simulink model "SF011A_EotLrng"  (R2013b)
settings: Solver=FixedStepDiscrete  SolverMode=SingleTasking  StartTime=0.0  StopTime=1  FixedStep=0.002  RelTol=1e-3
values from neighbouring files (symbols this model uses):
  ARCHGLBPRM_FLOATZEROTHD_ULS_F32 = DataDict.Constant    [SF011A_EotLrng_DataDict.m]
  CNVTOMILLISEC_MILLISECPERCNT_F32 = DataDict.Constant    [SF011A_EotLrng_DataDict.m]
  CORRLNFLT_CNT_U08 = DataDict.Constant    [SF011A_EotLrng_DataDict.m]
  DEBSTEP_CNT_U16 = DataDict.Constant    [SF011A_EotLrng_DataDict.m]
  EOTLIMDETD_CNT_LOGL = DataDict.Constant    [SF011A_EotLrng_DataDict.m]
  EOTLIMNOTDETD_CNT_LOGL = DataDict.Constant    [SF011A_EotLrng_DataDict.m]
  EotLrngAuthyStrtLrn = DataDict.Calibration    [SF011A_EotLrng_DataDict.m]
  EotLrngEotLrnTmr = DataDict.Calibration    [SF011A_EotLrng_DataDict.m]
  EotLrngHwAgOverTrvlCnt = DataDict.Calibration    [SF011A_EotLrng_DataDict.m]
  EotLrngHwAgOverTrvlEntr = DataDict.Calibration    [SF011A_EotLrng_DataDict.m]
  EotLrngHwAgOverTrvlExit = DataDict.Calibration    [SF011A_EotLrng_DataDict.m]
  EotLrngHwTqEotLrn = DataDict.Calibration    [SF011A_EotLrng_DataDict.m]
  EotLrngMotVelEotLrn = DataDict.Calibration    [SF011A_EotLrng_DataDict.m]
  EotLrngRackTrvlMax = DataDict.Calibration    [SF011A_EotLrng_DataDict.m]
  EotLrngRackTrvlMin = DataDict.Calibration    [SF011A_EotLrng_DataDict.m]
  EotLrngRstAuthyMin = DataDict.Calibration    [SF011A_EotLrng_DataDict.m]
  EotProtnRackTrvlLimrEna = DataDict.ImprtdCal    [SF011A_EotLrng_DataDict.m]
  HwAgOverTrvl = DataDict.NTC    [SF011A_EotLrng_DataDict.m]
  HWAGOVERTRVLMAXCNT_CNT_U08 = DataDict.Constant    [SF011A_EotLrng_DataDict.m]
  NODEBSTEP_CNT_U16 = DataDict.Constant    [SF011A_EotLrng_DataDict.m]
  OUTOFRNGFLT_CNT_U08 = DataDict.Constant    [SF011A_EotLrng_DataDict.m]
  RackEotStorgFlt = DataDict.NTC    [SF011A_EotLrng_DataDict.m]
  SIGAVLFLT_CNT_U08 = DataDict.Constant    [SF011A_EotLrng_DataDict.m]
undefined symbols (not defined in the file or in its folder): NtcSts1, NvmGetErrSts1, SigQlfr1
libraries: simulink x19, NxtrNvM x12, NxtrAbslt x5, NxtrLim x4, NxtrMax x3, NxtrMin x3
(part 3 of 7)

== system SF011A_EotLrng/EotLrng/EotLrngInit1/NvmNotVal ==
  Action Port : ActionPort  ActionType=then
  Cal1 : Constant  RequirementInfo="{'linktype_rmi_doors' '0000ba59 (/E-STEER Core/SubSystem Specifications/Application Functions/SF011A Learned EOT Limits)' '#SF011A_124' 'true' 'REQ:  SF011A_124' '' } %GIDa_035de4f9_96cc_4fa1_acd4_8bfcce4812e0"  Value=EotLrngRackTrvlMin
  Cal2 : Constant  RequirementInfo="{'linktype_rmi_doors' '0000ba59 (/E-STEER Core/SubSystem Specifications/Application Functions/SF011A Learned EOT Limits)' '#SF011A_124' 'true' 'REQ:  SF011A_124' '' } %GIDa_01b27a86_f72b_45a9_877f_2950e2d94a2a"  Value=EotLrngRackTrvlMin
  Constant1 : Constant  RequirementInfo="{'linktype_rmi_doors' '0000ba59 (/E-STEER Core/SubSystem Specifications/Application Functions/SF011A Learned EOT Limits)' '#SF011A_124' 'true' 'REQ:  SF011A_124' '' } %GIDa_1ebed793_de7b_4df7_85c2_e94d2e34449d"  Value=EOTLIMNOTDETD_CNT_LOGL
  Constant2 : Constant  RequirementInfo="{'linktype_rmi_doors' '0000ba59 (/E-STEER Core/SubSystem Specifications/Application Functions/SF011A Learned EOT Limits)' '#SF011A_124' 'true' 'REQ:  SF011A_124' '' } %GIDa_066674ad_e74a_483b_a55d_646f85c07109"  Value=EOTLIMNOTDETD_CNT_LOGL
  CopyRight2 : Subsystem  Description=|  mask(Copyright Information){none=on}
      | Copyright info block.                                               
      |                                                                     
      | Place copyright information at the top of every subsystem in design.
      mask prompts: none "No parameters"
      mask help: Place copyright information at the top of every subsystem in design.
      mask Display:
      | NxtrConf = 'Nexteer Confidential';
      | 
      | sys = bdroot; %handle for the current model ("system")
      | first = get_param(sys,'Created');
      | if(isempty(first))
      |     first = datestr(now,'yyyy');
      | else
      |     first = first(end-3:end);  %year is last four digits
      | end
      | 
      | last = get_param(sys,'LastModifiedDate');
      | if isempty(last)
      |     last = datestr(now,'yyyy');
      | else
      |     last = last(end-3:end);
      | end
      | 
      | if strcmp(first,last)
      |     fprintf('%s -- Copyright %s Nexteer',NxtrConf,first)
      | else
      |     fprintf('%s -- %s%s- %s Nexteer',NxtrConf,char(169),first,last)
      | end
  EotNotDetd : DataStoreWrite  RequirementInfo="{'linktype_rmi_doors' '0000ba59 (/E-STEER Core/SubSystem Specifications/Application Functions/SF011A Learned EOT Limits)' '#SF011A_124' 'true' 'REQ:  SF011A_124' '' } %GIDa_67ea3644_1ed5_47b1_a1b5_07943d39ffbc"  DataStoreName=EotNvmData  DataStoreElements=EotNvmData.CwEot#EotNvmData.CcwEot#EotNvmData.CwEotDetd#EotNvmData.CcwEotDetd
  Set Ram Block Status : NxtrNvM/Set Ram Block Status  RequirementInfo="{'linktype_rmi_doors' '0000ba59 (/E-STEER Core/SubSystem Specifications/Application Functions/SF011A Learned EOT Limits)' '#SF011A_124' 'true' 'REQ:  SF011A_124' '' } %GIDa_cd84de67_5aef_4c01_bda0_51f502c42aea"  FuncName=Set Ram Block Status  NvMBlockName=EotNvmData  VoidFuncRtn=on  BlockChanged_DSN=NvMSRBS_BlockChanged1  Return_DSN=NvMSRBS_Return1
      settings: AttributesFormatString=%<FuncName>
  Unary Minus : UnaryMinus  RequirementInfo="{'linktype_rmi_doors' '0000ba59 (/E-STEER Core/SubSystem Specifications/Application Functions/SF011A Learned EOT Limits)' '#SF011A_124' 'true' 'REQ:  SF011A_124' '' } %GIDa_d2217dbc_c775_4562_a13a_db7a1fc359c1"
  WriteFlag : Constant  RequirementInfo="{'linktype_rmi_doors' '0000ba59 (/E-STEER Core/SubSystem Specifications/Application Functions/SF011A Learned EOT Limits)' '#SF011A_124' 'true' 'REQ:  SF011A_124' '' } %GIDa_0fcbdb88_2c6a_4773_b445_1f58a3cfa24b"  OutDataTypeStr=boolean
      settings: AttributesFormatString=%<OutDataTypeStr>
  wires:
  Cal1/1 -> EotNotDetd/1
  Constant2/1 -> EotNotDetd/3
  Constant1/1 -> EotNotDetd/4
  Cal2/1 -> Unary Minus/1
  Unary Minus/1 -> EotNotDetd/2
  WriteFlag/1 -> Set Ram Block Status/1

== system SF011A_EotLrng/EotLrng/EotLrngInit1/RstEot ==
  note: 'ResetLimitRequest' is applicable only when SRL Enable is FALSE.
      | So 'IF' block is executed only when 'EotProtnRackTrvlLimrEna' is FALSE.
  Action Port : ActionPort  ActionType=then
  Cal1 : Constant  RequirementInfo="{'linktype_rmi_doors' '0000ba59 (/E-STEER Core/SubSystem Specifications/Application Functions/SF011A Learned EOT Limits)' '#SF011A_65' 'true' 'REQ:  SF011A_65' '' } %GIDa_8a14116a_f5ff_4f97_ae11_7182dd2cd95a"  Value=EotLrngRackTrvlMin
  Cal2 : Constant  RequirementInfo="{'linktype_rmi_doors' '0000ba59 (/E-STEER Core/SubSystem Specifications/Application Functions/SF011A Learned EOT Limits)' '#SF011A_66' 'true' 'REQ:  SF011A_66' '' } %GIDa_f5c0a088_5e82_430d_9c85_3e33e4dedd97"  Value=EotLrngRackTrvlMin
  Calibration4 : Constant  Value=EotProtnRackTrvlLimrEna
  ChkRstLimReq : Subsystem  RequirementInfo="{'linktype_rmi_doors' '0000ba59 (/E-STEER Core/SubSystem Specifications/Application Functions/SF011A Learned EOT Limits)' '#SF011A_120' 'true' 'REQ:  SF011A_120' '' } %GIDa_b83ed28f_298f_4fb9_b00a_69d67f564ffe"  TreatAsAtomicUnit=on
  Constant2 : Constant  RequirementInfo="{'linktype_rmi_doors' '0000ba59 (/E-STEER Core/SubSystem Specifications/Application Functions/SF011A Learned EOT Limits)' '#SF011A_67' 'true' 'REQ:  SF011A_67' '' } %GIDa_aa357eb7_da8e_4d45_9211_17e2d7de8510"  Value=EOTLIMNOTDETD_CNT_LOGL
  Constant3 : Constant  RequirementInfo="{'linktype_rmi_doors' '0000ba59 (/E-STEER Core/SubSystem Specifications/Application Functions/SF011A Learned EOT Limits)' '#SF011A_68' 'true' 'REQ:  SF011A_68' '' } %GIDa_8e713c15_fb38_440b_b663_257e60f908ef"  Value=EOTLIMNOTDETD_CNT_LOGL
  Copyright1 : Subsystem  Description=|  mask(Copyright Information){none=on}
      | Copyright info block.                                               
      |                                                                     
      | Place copyright information at the top of every subsystem in design.
      mask prompts: none "No parameters"
      mask help: Place copyright information at the top of every subsystem in design.
      mask Display:
      | NxtrConf = 'Nexteer Confidential';
      | 
      | sys = bdroot; %handle for the current model ("system")
      | first = get_param(sys,'Created');
      | if(isempty(first))
      |     first = datestr(now,'yyyy');
      | else
      |     first = first(end-3:end);  %year is last four digits
      | end
      | 
      | last = get_param(sys,'LastModifiedDate');
      | if isempty(last)
      |     last = datestr(now,'yyyy');
      | else
      |     last = last(end-3:end);
      | end
      | 
      | if strcmp(first,last)
      |     fprintf('%s\nCopyright  %s Nexteer',NxtrConf,first);
      | else
      |     fprintf('%s\n%s%s-%s Nexteer',NxtrConf,char(169),first,last);
      | end
  EotNotDetd : DataStoreWrite  RequirementInfo="{'linktype_rmi_doors' '0000ba59 (/E-STEER Core/SubSystem Specifications/Application Functions/SF011A Learned EOT Limits)' '#SF011A_65' 'true' 'REQ:  SF011A_65' '' ; 'linktype_rmi_doors' '0000ba59 (/E-STEER Core/SubSystem Specifications/Application Functions/SF011A Learned EOT Limits)' '#SF011A_66' 'true' 'REQ:  SF011A_66' '' ; 'linktype_rmi_doors' '0000ba59 (/E-STEER Core/SubSystem Specifications/Application Functions/SF011A Learned EOT Limits)' '#SF011A_67' 'true' 'REQ:  SF011A_67' '' ; 'linktype_rmi_doors' '0000ba59 (/E-STEER Core/SubSystem Specifications/Application Functions/SF011A Learned EOT Limits)' '#SF011A_68' 'true' 'REQ:  SF011A_68' '' } %GIDa_c154dafa_482c_4d0d_b49a_45c1c207fc69"  DataStoreName=EotNvmData  DataStoreElements=EotNvmData.CwEot#EotNvmData.CcwEot#EotNvmData.CwEotDetd#EotNvmData.CcwEotDetd
  If1 : If  IfExpression=~u1  ShowElse=off
  Unary Minus : UnaryMinus  RequirementInfo="{'linktype_rmi_doors' '0000ba59 (/E-STEER Core/SubSystem Specifications/Application Functions/SF011A Learned EOT Limits)' '#SF011A_66' 'true' 'REQ:  SF011A_66' '' } %GIDa_7d675248_4626_4542_a80b_dcf5738ed4de"
  wires:
  Cal1/1 -> EotNotDetd/1
  Constant2/1 -> EotNotDetd/3
  Constant3/1 -> EotNotDetd/4
  Cal2/1 -> Unary Minus/1
  Unary Minus/1 -> EotNotDetd/2
  Calibration4/1 -> If1/1
  If1/1 -> ChkRstLimReq/Action

== system SF011A_EotLrng/EotLrng/EotLrngInit1/SRLNotEna ==
  Action Port : ActionPort  ActionType=then
  CopyRight2 : Subsystem  Description=|  mask(Copyright Information){none=on}
      | Copyright info block.                                               
      |                                                                     
      | Place copyright information at the top of every subsystem in design.
      mask prompts: none "No parameters"
      mask help: Place copyright information at the top of every subsystem in design.
      mask Display:
      | NxtrConf = 'Nexteer Confidential';
      | 
      | sys = bdroot; %handle for the current model ("system")
      | first = get_param(sys,'Created');
      | if(isempty(first))
      |     first = datestr(now,'yyyy');
      | else
      |     first = first(end-3:end);  %year is last four digits
      | end
      | 
      | last = get_param(sys,'LastModifiedDate');
      | if isempty(last)
      |     last = datestr(now,'yyyy');
      | else
      |     last = last(end-3:end);
      | end
      | 
      | if strcmp(first,last)
      |     fprintf('%s -- Copyright %s Nexteer',NxtrConf,first)
      | else
      |     fprintf('%s -- %s%s- %s Nexteer',NxtrConf,char(169),first,last)
      | end
  Data Store Write1 : DataStoreWrite  RequirementInfo="{'linktype_rmi_doors' '0000ba59 (/E-STEER Core/SubSystem Specifications/Application Functions/SF011A Learned EOT Limits)' '#SF011A_125' 'true' 'REQ:  SF011A_125' '' } %GIDa_d378e069_f629_4d72_894b_869d827cea0f"  DataStoreName=CwEotRefTmr
  Data Store Write2 : DataStoreWrite  RequirementInfo="{'linktype_rmi_doors' '0000ba59 (/E-STEER Core/SubSystem Specifications/Application Functions/SF011A Learned EOT Limits)' '#SF011A_125' 'true' 'REQ:  SF011A_125' '' } %GIDa_c50f2ed6_18b8_4a79_9256_efd4e1cd0e04"  DataStoreName=CcwEotRefTmr
  GetRefTmr100MicroSec32bit : Subsystem  RequirementInfo="{'linktype_rmi_doors' '0000ba59 (/E-STEER Core/SubSystem Specifications/Application Functions/SF011A Learned EOT Limits)' '#SF011A_125' 'true' 'REQ:  SF011A_125' '' } %GIDa_8d57e8b2_6972_45c8_8aed_33e94bb589a0"
  Set Ram Block Status : NxtrNvM/Set Ram Block Status  RequirementInfo="{'linktype_rmi_doors' '0000ba59 (/E-STEER Core/SubSystem Specifications/Application Functions/SF011A Learned EOT Limits)' '#SF011A_71' 'true' 'REQ:  SF011A_71' '' } %GIDa_8d0a3400_ce1c_4c12_9bc7_eab84e420ace"  FuncName=Set Ram Block Status  NvMBlockName=EotNvmData  VoidFuncRtn=on  BlockChanged_DSN=NvMSRBS_BlockChanged2  Return_DSN=NvMSRBS_Return2
      settings: AttributesFormatString=%<FuncName>
  WriteFlag : Constant  RequirementInfo="{'linktype_rmi_doors' '0000ba59 (/E-STEER Core/SubSystem Specifications/Application Functions/SF011A Learned EOT Limits)' '#SF011A_71' 'true' 'REQ:  SF011A_71' '' } %GIDa_d9597664_5da8_4eef_8b58_6fe14386c65c"  OutDataTypeStr=boolean
      settings: AttributesFormatString=%<OutDataTypeStr>
  wires:
  GetRefTmr100MicroSec32bit/1(RefTmr) -> Data Store Write2/1, Data Store Write1/1
  WriteFlag/1 -> Set Ram Block Status/1

== system SF011A_EotLrng/EotLrng/EotLrngInit1/SetOverTrvlDiagcPass ==
  NtcNr : Inport
  NtcStInfo : Inport  Port=2
  NtcSts : Inport  Port=3
  DebStep : Inport  Port=4
  SetNtcSts : Subsystem  RequirementInfo={} %GIDa_9e323aaf_8c1e_43be_a15a_0107c73abfe9  TreatAsAtomicUnit=on
      settings: RTWSystemCode=Inline
  wires:
  NtcNr/1 -> SetNtcSts/1(NtcNr)  "NtcNr"
  NtcSts/1 -> SetNtcSts/3(NtcSts)
  DebStep/1 -> SetNtcSts/4(DebStep)
  NtcStInfo/1 -> SetNtcSts/2(NtcStInfo)

== system SF011A_EotLrng/EotLrng/EotLrngPer1/CopyRight2 ==

== system SF011A_EotLrng/EotLrng/EotLrngPer1/HwAgCwAndCcwMax ==
  HwAg : Inport  RequirementInfo={} %GIDa_58741c58_0ee8_47f7_8539_fc4bf25b9bfb
  HwAgAuthy : Inport  RequirementInfo="{'linktype_rmi_doors' '0000ba59 (/E-STEER Core/SubSystem Specifications/Application Functions/SF011A Learned EOT Limits)' '#SF011A_156' 'true' 'REQ:  SF011A_156' '' ; 'linktype_rmi_doors' '0000ba59 (/E-STEER Core/SubSystem Specifications/Application Functions/SF011A Learned EOT Limits)' '#SF011A_158' 'true' 'REQ:  SF011A_158' '' } %GIDa_fbd8c566_5363_4a96_8e79_d2f0f22f358c"  Port=2
  HwAgCwDetd : Inport  RequirementInfo={} %GIDa_42146e60_6491_4cfb_867f_f1091c71a37f  Port=3
  HwAgCcwDetd : Inport  RequirementInfo={} %GIDa_3f214823_f21d_45f8_844e_ba7a8ea07747  Port=4
  Conf : Sum  RequirementInfo="{'linktype_rmi_doors' '0000ba59 (/E-STEER Core/SubSystem Specifications/Application Functions/SF011A Learned EOT Limits)' '#SF011A_145' 'true' 'REQ:  SF011A_145' '' ; 'linktype_rmi_doors' '0000ba59 (/E-STEER Core/SubSystem Specifications/Application Functions/SF011A Learned EOT Limits)' '#SF011A_156' 'true' 'REQ:  SF011A_156' '' ; 'linktype_rmi_doors' '0000ba59 (/E-STEER Core/SubSystem Specifications/Application Functions/SF011A Learned EOT Limits)' '#SF011A_158' 'true' 'REQ:  SF011A_158' '' } %GIDa_bf8efe5e_d1fb_49c5_9ca8_3a5e9fe4b02d"  Inputs=+-
  Constant : Constant  RequirementInfo="{'linktype_rmi_doors' '0000ba59 (/E-STEER Core/SubSystem Specifications/Application Functions/SF011A Learned EOT Limits)' '#SF011A_156' 'true' 'REQ:  SF011A_156' '' ; 'linktype_rmi_doors' '0000ba59 (/E-STEER Core/SubSystem Specifications/Application Functions/SF011A Learned EOT Limits)' '#SF011A_158' 'true' 'REQ:  SF011A_158' '' } %GIDa_0eba6ba2_6b16_45eb_a7cf_ae1f1a9ed1c4"  OutDataTypeStr=single
      settings: AttributesFormatString=%<OutDataTypeStr>
  Constant4 : Constant  RequirementInfo="{'linktype_rmi_doors' '0000ba59 (/E-STEER Core/SubSystem Specifications/Application Functions/SF011A Learned EOT Limits)' '#SF011A_156' 'true' 'REQ:  SF011A_156' '' ; 'linktype_rmi_doors' '0000ba59 (/E-STEER Core/SubSystem Specifications/Application Functions/SF011A Learned EOT Limits)' '#SF011A_158' 'true' 'REQ:  SF011A_158' '' } %GIDa_d72fb292_81de_491b_ad99_a4a5661cf7d7"  Value=ARCHGLBPRM_FLOATZEROTHD_ULS_F32
  CopyRight2 : Subsystem  Description=|  mask(Copyright Information){none=on}
      | Copyright info block.                                               
      |                                                                     
      | Place copyright information at the top of every subsystem in design.
      mask prompts: none "No parameters"
      mask help: Place copyright information at the top of every subsystem in design.
      mask Display:
      | NxtrConf = 'Nexteer Confidential';
      | 
      | sys = bdroot; %handle for the current model ("system")
      | first = get_param(sys,'Created');
      | if(isempty(first))
      |     first = datestr(now,'yyyy');
      | else
      |     first = first(end-3:end);  %year is last four digits
      | end
      | 
      | last = get_param(sys,'LastModifiedDate');
      | if isempty(last)
      |     last = datestr(now,'yyyy');
      | else
      |     last = last(end-3:end);
      | end
      | 
      | if strcmp(first,last)
      |     fprintf('%s -- Copyright %s Nexteer',NxtrConf,first)
      | else
      |     fprintf('%s -- %s%s- %s Nexteer',NxtrConf,char(169),first,last)
      | end
  HwAgCwAndCcw : Subsystem  RequirementInfo="{'linktype_rmi_doors' '0000ba59 (/E-STEER Core/SubSystem Specifications/Application Functions/SF011A Learned EOT Limits)' '#SF011A_158' 'true' 'REQ:  SF011A_158' '' } %GIDa_77bc3317_1f5b_4708_9123_1bb25581bbdf"  TreatAsAtomicUnit=on
  If : If  RequirementInfo="{'linktype_rmi_doors' '0000ba59 (/E-STEER Core/SubSystem Specifications/Application Functions/SF011A Learned EOT Limits)' '#SF011A_156' 'true' 'REQ:  SF011A_156' '' ; 'linktype_rmi_doors' '0000ba59 (/E-STEER Core/SubSystem Specifications/Application Functions/SF011A Learned EOT Limits)' '#SF011A_158' 'true' 'REQ:  SF011A_158' '' } %GIDa_feff3a4a_5231_4460_af4d_ff321ace2938"  IfExpression=u1  ShowElse=off
  Relational Operator1 : RelationalOperator  RequirementInfo="{'linktype_rmi_doors' '0000ba59 (/E-STEER Core/SubSystem Specifications/Application Functions/SF011A Learned EOT Limits)' '#SF011A_156' 'true' 'REQ:  SF011A_156' '' ; 'linktype_rmi_doors' '0000ba59 (/E-STEER Core/SubSystem Specifications/Application Functions/SF011A Learned EOT Limits)' '#SF011A_158' 'true' 'REQ:  SF011A_158' '' } %GIDa_5f57789c_cdb5_4887_9bd9_e5225cc82d4e"  Operator=<  OutDataTypeStr=boolean
  wires:
  HwAg/1 -> HwAgCwAndCcw/1(HwAg)
  Conf/1 -> Relational Operator1/1
  Constant4/1 -> Relational Operator1/2
  Relational Operator1/1 -> If/1
  If/1 -> HwAgCwAndCcw/Action
  Constant/1 -> Conf/1
  HwAgAuthy/1 -> Conf/2
  HwAgCwDetd/1 -> HwAgCwAndCcw/2(HwAgCwDetd)
  HwAgCcwDetd/1 -> HwAgCwAndCcw/3(HwAgCcwDetd)

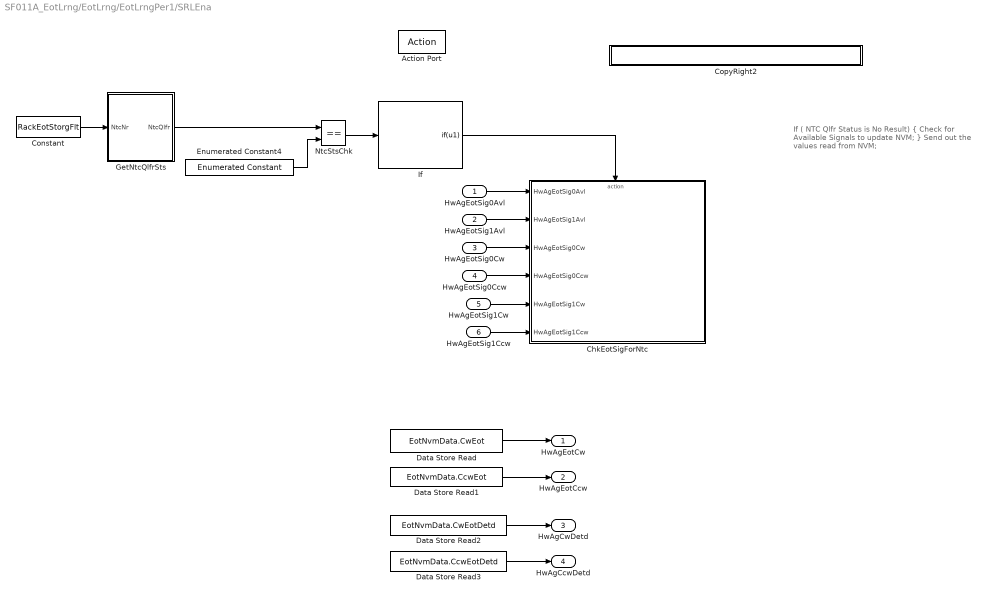
== system SF011A_EotLrng/EotLrng/EotLrngPer1/SRLEna ==
  note: If ( NTC Qlfr Status is No Result)
      | {
      | 	Check for Available Signals to update NVM;
      | }
      |
      | Send out the values read from NVM;
  HwAgEotSig0Avl : Inport
  HwAgEotSig1Avl : Inport  Port=2
  HwAgEotSig0Cw : Inport  Port=3
  HwAgEotSig0Ccw : Inport  Port=4
  HwAgEotSig1Cw : Inport  Port=5
  HwAgEotSig1Ccw : Inport  Port=6
  Action Port : ActionPort  ActionType=else
  ChkEotSigForNtc : Subsystem  Priority=2  TreatAsAtomicUnit=on
  Constant : Constant  Value=RackEotStorgFlt
  CopyRight2 : Subsystem  Description=|  mask(Copyright Information){none=on}
      | Copyright info block.                                               
      |                                                                     
      | Place copyright information at the top of every subsystem in design.
      mask prompts: none "No parameters"
      mask help: Place copyright information at the top of every subsystem in design.
      mask Display:
      | NxtrConf = 'Nexteer Confidential';
      | 
      | sys = bdroot; %handle for the current model ("system")
      | first = get_param(sys,'Created');
      | if(isempty(first))
      |     first = datestr(now,'yyyy');
      | else
      |     first = first(end-3:end);  %year is last four digits
      | end
      | 
      | last = get_param(sys,'LastModifiedDate');
      | if isempty(last)
      |     last = datestr(now,'yyyy');
      | else
      |     last = last(end-3:end);
      | end
      | 
      | if strcmp(first,last)
      |     fprintf('%s -- Copyright %s Nexteer',NxtrConf,first)
      | else
      |     fprintf('%s -- %s%s- %s Nexteer',NxtrConf,char(169),first,last)
      | end
  Data Store Read : DataStoreRead  RequirementInfo="{'linktype_rmi_doors' '0000ba59 (/E-STEER Core/SubSystem Specifications/Application Functions/SF011A Learned EOT Limits)' '#SF011A_151' 'true' 'REQ:  SF011A_151' '' } %GIDa_491bb231_a96c_471a_a0b1_cb46d3ab7fd8"  DataStoreName=EotNvmData  DataStoreElements=EotNvmData.CwEot
  Data Store Read1 : DataStoreRead  RequirementInfo="{'linktype_rmi_doors' '0000ba59 (/E-STEER Core/SubSystem Specifications/Application Functions/SF011A Learned EOT Limits)' '#SF011A_151' 'true' 'REQ:  SF011A_151' '' } %GIDa_e22716e1_ea90_4526_a8a2_524f602455ba"  DataStoreName=EotNvmData  DataStoreElements=EotNvmData.CcwEot
  Data Store Read2 : DataStoreRead  RequirementInfo="{'linktype_rmi_doors' '0000ba59 (/E-STEER Core/SubSystem Specifications/Application Functions/SF011A Learned EOT Limits)' '#SF011A_152' 'true' 'REQ:  SF011A_152' '' } %GIDa_803dbdde_f1bc_4dcd_811b_135296056d76"  DataStoreName=EotNvmData  DataStoreElements=EotNvmData.CwEotDetd
  Data Store Read3 : DataStoreRead  RequirementInfo="{'linktype_rmi_doors' '0000ba59 (/E-STEER Core/SubSystem Specifications/Application Functions/SF011A Learned EOT Limits)' '#SF011A_152' 'true' 'REQ:  SF011A_152' '' } %GIDa_81638686_3894_4a3b_89e5_bc8caeb35295"  DataStoreName=EotNvmData  DataStoreElements=EotNvmData.CcwEotDetd
  Enumerated Constant4 : simulink/Sources/Enumerated Constant  RequirementInfo="{'linktype_rmi_doors' '0000ba59 (/E-STEER Core/SubSystem Specifications/Application Functions/SF011A Learned EOT Limits)' '#SF011A_144' 'true' 'REQ:  SF011A_144' '' } %GIDa_d54fdf58_b16f_405c_be57_dbc33b57e03e"  OutDataTypeStr=Enum: SigQlfr1  Value=SigQlfr1.SIGQLFR_NORES  SampleTime=inf
  GetNtcQlfrSts : Subsystem  RequirementInfo="{'linktype_rmi_doors' '0000ba59 (/E-STEER Core/SubSystem Specifications/Application Functions/SF011A Learned EOT Limits)' '#SF011A_144' 'true' 'REQ:  SF011A_144' '' } %GIDa_4c60277e_e0ab_4449_8203_11119612fe69"  Priority=0  TreatAsAtomicUnit=on  mask(GetNTC){}
      mask help: GetNTC library block
      settings: RTWSystemCode=Inline
  If : If  RequirementInfo="{'linktype_rmi_doors' '0000ba59 (/E-STEER Core/SubSystem Specifications/Application Functions/SF011A Learned EOT Limits)' '#SF011A_144' 'true' 'REQ:  SF011A_144' '' } %GIDa_00dfac98_a167_441c_a0ad_0ab30e5da204"  Priority=1  IfExpression=u1  ShowElse=off
  NtcStsChk : RelationalOperator  RequirementInfo="{'linktype_rmi_doors' '0000ba59 (/E-STEER Core/SubSystem Specifications/Application Functions/SF011A Learned EOT Limits)' '#SF011A_144' 'true' 'REQ:  SF011A_144' '' } %GIDa_ddf88f27_8f18_4c5d_9adb_9f4c149e8d0b"  Operator===  OutDataTypeStr=boolean
  HwAgEotCw : Outport  RequirementInfo="{'linktype_rmi_doors' '0000ba59 (/E-STEER Core/SubSystem Specifications/Application Functions/SF011A Learned EOT Limits)' '#SF011A_151' 'true' 'REQ:  SF011A_151' '' } %GIDa_fda7daf0_aaae_4096_9ebe_71b9db7e29f8"
  HwAgEotCcw : Outport  RequirementInfo="{'linktype_rmi_doors' '0000ba59 (/E-STEER Core/SubSystem Specifications/Application Functions/SF011A Learned EOT Limits)' '#SF011A_151' 'true' 'REQ:  SF011A_151' '' } %GIDa_84ec16c1_5dae_46bb_8c56_2a910f1f9ddc"  Port=2
  HwAgCwDetd : Outport  RequirementInfo="{'linktype_rmi_doors' '0000ba59 (/E-STEER Core/SubSystem Specifications/Application Functions/SF011A Learned EOT Limits)' '#SF011A_152' 'true' 'REQ:  SF011A_152' '' } %GIDa_67f65cbe_992b_48c5_9d00_546aabda8cbc"  Port=3
  HwAgCcwDetd : Outport  RequirementInfo="{'linktype_rmi_doors' '0000ba59 (/E-STEER Core/SubSystem Specifications/Application Functions/SF011A Learned EOT Limits)' '#SF011A_152' 'true' 'REQ:  SF011A_152' '' } %GIDa_23fcd4ad_b638_4e85_88df_027c5135ac77"  Port=4
  wires:
  Constant/1 -> GetNtcQlfrSts/1(NtcNr)
  Enumerated Constant4/1 -> NtcStsChk/2
  NtcStsChk/1 -> If/1
  HwAgEotSig0Avl/1 -> ChkEotSigForNtc/1(HwAgEotSig0Avl)
  HwAgEotSig1Avl/1 -> ChkEotSigForNtc/2(HwAgEotSig1Avl)
  HwAgEotSig0Cw/1 -> ChkEotSigForNtc/3(HwAgEotSig0Cw)
  HwAgEotSig0Ccw/1 -> ChkEotSigForNtc/4(HwAgEotSig0Ccw)
  HwAgEotSig1Cw/1 -> ChkEotSigForNtc/5(HwAgEotSig1Cw)
  HwAgEotSig1Ccw/1 -> ChkEotSigForNtc/6(HwAgEotSig1Ccw)
  If/1 -> ChkEotSigForNtc/Action
  GetNtcQlfrSts/1(NtcQlfr) -> NtcStsChk/1
  Data Store Read2/1 -> HwAgCwDetd/1
  Data Store Read3/1 -> HwAgCcwDetd/1
  Data Store Read/1 -> HwAgEotCw/1
  Data Store Read1/1 -> HwAgEotCcw/1

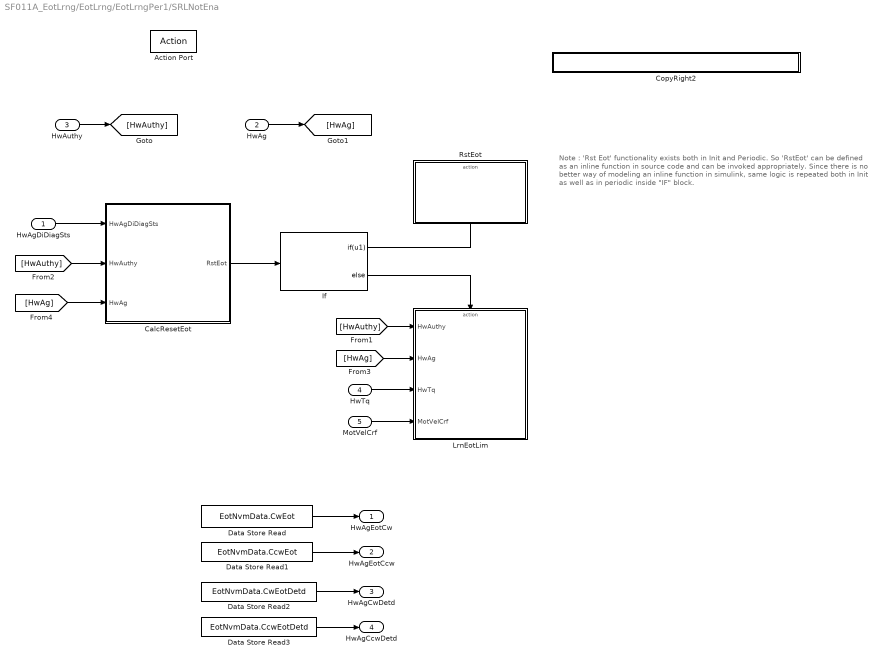
== system SF011A_EotLrng/EotLrng/EotLrngPer1/SRLNotEna ==
  note: Note : 'Rst Eot' functionality exists both in Init and Periodic.
      | So 'RstEot' can be defined as an inline function in source code and can be invoked
      | appropriately. Since there is no better way of modeling an inline function in simulink,
      | same logic is repeated both in Init as well as in periodic inside "IF" block.
  HwAgDiDiagSts : Inport
  HwAg : Inport  Port=2
  HwAuthy : Inport  Port=3
  HwTq : Inport  Port=4
  MotVelCrf : Inport  Port=5
  Action Port : ActionPort  ActionType=then
  CalcResetEot : Subsystem  Priority=0  TreatAsAtomicUnit=on
  CopyRight2 : Subsystem  Description=|  mask(Copyright Information){none=on}
      | Copyright info block.                                               
      |                                                                     
      | Place copyright information at the top of every subsystem in design.
      mask prompts: none "No parameters"
      mask help: Place copyright information at the top of every subsystem in design.
      mask Display:
      | NxtrConf = 'Nexteer Confidential';
      | 
      | sys = bdroot; %handle for the current model ("system")
      | first = get_param(sys,'Created');
      | if(isempty(first))
      |     first = datestr(now,'yyyy');
      | else
      |     first = first(end-3:end);  %year is last four digits
      | end
      | 
      | last = get_param(sys,'LastModifiedDate');
      | if isempty(last)
      |     last = datestr(now,'yyyy');
      | else
      |     last = last(end-3:end);
      | end
      | 
      | if strcmp(first,last)
      |     fprintf('%s -- Copyright %s Nexteer',NxtrConf,first)
      | else
      |     fprintf('%s -- %s%s- %s Nexteer',NxtrConf,char(169),first,last)
      | end
  Data Store Read : DataStoreRead  RequirementInfo="{'linktype_rmi_doors' '0000ba59 (/E-STEER Core/SubSystem Specifications/Application Functions/SF011A Learned EOT Limits)' '#SF011A_152' 'true' 'REQ:  SF011A_152' '' } %GIDa_e6e4a090_8f56_4550_9411_905043d89ec9"  DataStoreName=EotNvmData  DataStoreElements=EotNvmData.CwEot
  Data Store Read1 : DataStoreRead  RequirementInfo="{'linktype_rmi_doors' '0000ba59 (/E-STEER Core/SubSystem Specifications/Application Functions/SF011A Learned EOT Limits)' '#SF011A_152' 'true' 'REQ:  SF011A_152' '' } %GIDa_57f7b2c9_ce66_4e64_aa00_2e33be35bf96"  DataStoreName=EotNvmData  DataStoreElements=EotNvmData.CcwEot
  Data Store Read2 : DataStoreRead  RequirementInfo="{'linktype_rmi_doors' '0000ba59 (/E-STEER Core/SubSystem Specifications/Application Functions/SF011A Learned EOT Limits)' '#SF011A_152' 'true' 'REQ:  SF011A_152' '' } %GIDa_1c8ac1be_b2fe_42d3_9f1e_87bea7bc78f5"  DataStoreName=EotNvmData  DataStoreElements=EotNvmData.CwEotDetd
  Data Store Read3 : DataStoreRead  RequirementInfo="{'linktype_rmi_doors' '0000ba59 (/E-STEER Core/SubSystem Specifications/Application Functions/SF011A Learned EOT Limits)' '#SF011A_152' 'true' 'REQ:  SF011A_152' '' } %GIDa_fbf998d0_abbd_4e2e_9173_7ac660a7097a"  DataStoreName=EotNvmData  DataStoreElements=EotNvmData.CcwEotDetd
  If : If  RequirementInfo="{'linktype_rmi_doors' '0000ba59 (/E-STEER Core/SubSystem Specifications/Application Functions/SF011A Learned EOT Limits)' '#SF011A_77' 'true' 'REQ:  SF011A_77' '' } %GIDa_0aa79ea6_77ec_4eb1_817b_135a8ab293c6"  Priority=1  IfExpression=u1
  LrnEotLim : Subsystem  TreatAsAtomicUnit=on
  RstEot : Subsystem  RequirementInfo="{'linktype_rmi_doors' '0000ba59 (/E-STEER Core/SubSystem Specifications/Application Functions/SF011A Learned EOT Limits)' '#SF011A_64' 'true' 'REQ:  SF011A_64' '' ; 'linktype_rmi_doors' '0000ba59 (/E-STEER Core/SubSystem Specifications/Application Functions/SF011A Learned EOT Limits)' '#SF011A_77' 'true' 'REQ:  SF011A_77' '' } %GIDa_52c91bf7_5122_422c_9233_27632b93939a"  TreatAsAtomicUnit=on
  HwAgEotCw : Outport  RequirementInfo="{'linktype_rmi_doors' '0000ba59 (/E-STEER Core/SubSystem Specifications/Application Functions/SF011A Learned EOT Limits)' '#SF011A_152' 'true' 'REQ:  SF011A_152' '' } %GIDa_f2d57ba9_aa8d_479c_9cc8_16e180750fa0"
  HwAgEotCcw : Outport  RequirementInfo="{'linktype_rmi_doors' '0000ba59 (/E-STEER Core/SubSystem Specifications/Application Functions/SF011A Learned EOT Limits)' '#SF011A_152' 'true' 'REQ:  SF011A_152' '' } %GIDa_27db5f88_6347_4271_b0df_6a54758f3e06"  Port=2
  HwAgCwDetd : Outport  RequirementInfo="{'linktype_rmi_doors' '0000ba59 (/E-STEER Core/SubSystem Specifications/Application Functions/SF011A Learned EOT Limits)' '#SF011A_152' 'true' 'REQ:  SF011A_152' '' } %GIDa_b05d0ec9_37ec_4da9_bb3b_3c23aee6b93b"  Port=3
  HwAgCcwDetd : Outport  RequirementInfo="{'linktype_rmi_doors' '0000ba59 (/E-STEER Core/SubSystem Specifications/Application Functions/SF011A Learned EOT Limits)' '#SF011A_152' 'true' 'REQ:  SF011A_152' '' } %GIDa_425014ec_6d0c_4dba_84fc_301e2e49fc38"  Port=4
  wires:
  HwAuthy/1 -> [HwAuthy]
  If/1 -> RstEot/Action
  HwAgDiDiagSts/1 -> CalcResetEot/1(HwAgDiDiagSts)
  [HwAg] -> CalcResetEot/3(HwAg)
  CalcResetEot/1(RstEot) -> If/1
  [HwAuthy] -> CalcResetEot/2(HwAuthy)
  If/2 -> LrnEotLim/Action
  HwTq/1 -> LrnEotLim/3(HwTq)
  MotVelCrf/1 -> LrnEotLim/4(MotVelCrf)
  [HwAuthy] -> LrnEotLim/1(HwAuthy)
  HwAg/1 -> [HwAg]
  [HwAg] -> LrnEotLim/2(HwAg)
  Data Store Read2/1 -> HwAgCwDetd/1
  Data Store Read3/1 -> HwAgCcwDetd/1
  Data Store Read/1 -> HwAgEotCw/1
  Data Store Read1/1 -> HwAgEotCcw/1

== system SF011A_EotLrng/EotLrng/GetHwAgOverTrvlCnt/CopyRight2 ==

== system SF011A_EotLrng/EotLrng/RstHwAgOverTrvlCnt/CopyRight2 ==

== system SF011A_EotLrng/EotLrng/RstMaxHwAgCwAndCcw/CopyRight2 ==

== system SF011A_EotLrng/EotLrng/RtnMaxHwAgCwAndCcw/CopyRight2 ==

== system SF011A_EotLrng/EotLrng/SerlComRstEot/CopyRight2 ==

== system SF011A_EotLrng/EotLrng/SerlComRstEot/SetRstLimReq ==
  Action Port : ActionPort  ActionType=then
  Constant : Constant  RequirementInfo="{'linktype_rmi_doors' '0000ba59 (/E-STEER Core/SubSystem Specifications/Application Functions/SF011A Learned EOT Limits)' '#SF011A_123' 'true' 'REQ:  SF011A_123' '' } %GIDa_80072151_4aff_45b9_8875_461114410ad3"  Value=true  OutDataTypeStr=boolean
      settings: AttributesFormatString=%<OutDataTypeStr>
  CopyRight2 : Subsystem  Description=|  mask(Copyright Information){none=on}
      | Copyright info block.                                               
      |                                                                     
      | Place copyright information at the top of every subsystem in design.
      mask prompts: none "No parameters"
      mask help: Place copyright information at the top of every subsystem in design.
      mask Display:
      | NxtrConf = 'Nexteer Confidential';
      | 
      | sys = bdroot; %handle for the current model ("system")
      | first = get_param(sys,'Created');
      | if(isempty(first))
      |     first = datestr(now,'yyyy');
      | else
      |     first = first(end-3:end);  %year is last four digits
      | end
      | 
      | last = get_param(sys,'LastModifiedDate');
      | if isempty(last)
      |     last = datestr(now,'yyyy');
      | else
      |     last = last(end-3:end);
      | end
      | 
      | if strcmp(first,last)
      |     fprintf('%s -- Copyright %s Nexteer',NxtrConf,first)
      | else
      |     fprintf('%s -- %s%s- %s Nexteer',NxtrConf,char(169),first,last)
      | end
  Update PIM3 : DataStoreWrite  RequirementInfo="{'linktype_rmi_doors' '0000ba59 (/E-STEER Core/SubSystem Specifications/Application Functions/SF011A Learned EOT Limits)' '#SF011A_123' 'true' 'REQ:  SF011A_123' '' } %GIDa_a977ed3a_c109_468e_8bf0_813090a9fca0"  DataStoreName=RstLimReq
  wires:
  Constant/1 -> Update PIM3/1

== system SF011A_EotLrng/EotLrng/SetHwAgOverTrvlCnt/CopyRight2 ==

== system SF011A_EotLrng/EotLrng/EotLrngInit1/NvmNotOk/CopyRight2 ==

== system SF011A_EotLrng/EotLrng/EotLrngInit1/NvmNotVal/CopyRight2 ==

== system SF011A_EotLrng/EotLrng/EotLrngInit1/RstEot/ChkRstLimReq ==
  Action Port : ActionPort  ActionType=then
  CopyRight2 : Subsystem  Description=|  mask(Copyright Information){none=on}
      | Copyright info block.                                               
      |                                                                     
      | Place copyright information at the top of every subsystem in design.
      mask prompts: none "No parameters"
      mask help: Place copyright information at the top of every subsystem in design.
      mask Display:
      | NxtrConf = 'Nexteer Confidential';
      | 
      | sys = bdroot; %handle for the current model ("system")
      | first = get_param(sys,'Created');
      | if(isempty(first))
      |     first = datestr(now,'yyyy');
      | else
      |     first = first(end-3:end);  %year is last four digits
      | end
      | 
      | last = get_param(sys,'LastModifiedDate');
      | if isempty(last)
      |     last = datestr(now,'yyyy');
      | else
      |     last = last(end-3:end);
      | end
      | 
      | if strcmp(first,last)
      |     fprintf('%s -- Copyright %s Nexteer',NxtrConf,first)
      | else
      |     fprintf('%s -- %s%s- %s Nexteer',NxtrConf,char(169),first,last)
      | end
  Data Store Read4 : DataStoreRead  RequirementInfo="{'linktype_rmi_doors' '0000ba59 (/E-STEER Core/SubSystem Specifications/Application Functions/SF011A Learned EOT Limits)' '#SF011A_120' 'true' 'REQ:  SF011A_120' '' } %GIDa_bbdcaebb_aa54_4c32_aceb_dfb7e5459836"  DataStoreName=RstLimReq
  If : If  RequirementInfo="{'linktype_rmi_doors' '0000ba59 (/E-STEER Core/SubSystem Specifications/Application Functions/SF011A Learned EOT Limits)' '#SF011A_120' 'true' 'REQ:  SF011A_120' '' } %GIDa_0c4f3b6a_a79f_4beb_a24b_d33f2f2aabe0"  IfExpression=u1  ShowElse=off
  ResetLimReq : Subsystem  RequirementInfo="{'linktype_rmi_doors' '0000ba59 (/E-STEER Core/SubSystem Specifications/Application Functions/SF011A Learned EOT Limits)' '#SF011A_120' 'true' 'REQ:  SF011A_120' '' } %GIDa_2dbe23da_3ce9_4548_9ac3_4137e2e9edeb"  TreatAsAtomicUnit=on
  wires:
  Data Store Read4/1 -> If/1
  If/1 -> ResetLimReq/Action

== system SF011A_EotLrng/EotLrng/EotLrngInit1/RstEot/Copyright1 ==

== system SF011A_EotLrng/EotLrng/EotLrngInit1/SRLNotEna/CopyRight2 ==

== system SF011A_EotLrng/EotLrng/EotLrngInit1/SRLNotEna/GetRefTmr100MicroSec32bit ==
  note: 1 count = 100 uSec
  note: seconds
  note: microseconds
  note: counts
  note: Wrap-to-zero
  note: GetRefTmr100MicroSec32bit
  CopyRight2 : Subsystem  Description=|  mask(Copyright Information){none=on}
      | Copyright info block.                                               
      |                                                                     
      | Place copyright information at the top of every subsystem in design.
      mask prompts: none "No parameters"
      mask help: Place copyright information at the top of every subsystem in design.
      mask Display:
      | NxtrConf = 'Nexteer Confidential';
      | 
      | sys = bdroot; %handle for the current model ("system")
      | first = get_param(sys,'Created');
      | if(isempty(first))
      |     first = datestr(now,'yyyy');
      | else
      |     first = first(end-3:end);  %year is last four digits
      | end
      | 
      | last = get_param(sys,'LastModifiedDate');
      | if isempty(last)
      |     last = datestr(now,'yyyy');
      | else
      |     last = last(end-3:end);
      | end
      | 
      | if strcmp(first,last)
      |     fprintf('%s -- Copyright %s Nexteer',NxtrConf,first)
      | else
      |     fprintf('%s -- %s%s- %s Nexteer',NxtrConf,char(169),first,last)
      | end
  Count per uSec : Constant  Value=0.01
  Data Store Read1 : DataStoreRead  DataStoreName=SimnTi
  Data Type Conversion1 : DataTypeConversion  OutDataTypeStr=uint32
  Divide1 : Product  Inputs=**
  Divide2 : Product  Inputs=*/
  Max Counts : Constant  Value=2^32-1
  Product1 : Product
  Product2 : Product
  Rounding : Rounding
  Subtract1 : Sum  Inputs=+-
  uSec per Sec : Constant  Value=1000000
  RefTmr : Outport
  wires:
  Product2/1 -> Subtract1/2
  Subtract1/1 -> Data Type Conversion1/1
  Rounding/1 -> Product2/1
  Divide2/1 -> Rounding/1
  Max Counts/1 -> Divide2/2, Product2/2
  Divide1/1 -> Divide2/1, Subtract1/1
  Product1/1 -> Divide1/1
  Data Store Read1/1 -> Product1/1
  Count per uSec/1 -> Divide1/2
  uSec per Sec/1 -> Product1/2
  Data Type Conversion1/1 -> RefTmr/1

== system SF011A_EotLrng/EotLrng/EotLrngInit1/SetOverTrvlDiagcPass/SetNtcSts ==
  note: Note:
      |
      | - "ISO Fault Debounce Design" Simulink block intent to use here for Simulation purpose only. Do not Code this block
  NtcNr : Inport
  NtcStInfo : Inport  Port=2
  NtcSts : Inport  Port=3
  DebStep : Inport  Port=4
  CopyRight2 : Subsystem  Description=|  mask(Copyright Information){none=on}
      | Copyright info block.                                               
      |                                                                     
      | Place copyright information at the top of every subsystem in design.
      mask prompts: none "No parameters"
      mask help: Place copyright information at the top of every subsystem in design.
      mask Display:
      | NxtrConf = 'Nexteer Confidential';
      | 
      | sys = bdroot; %handle for the current model ("system")
      | first = get_param(sys,'Created');
      | if(isempty(first))
      |     first = datestr(now,'yyyy');
      | else
      |     first = first(end-3:end);  %year is last four digits
      | end
      | 
      | last = get_param(sys,'LastModifiedDate');
      | if isempty(last)
      |     last = datestr(now,'yyyy');
      | else
      |     last = last(end-3:end);
      | end
      | 
      | if strcmp(first,last)
      |     fprintf('%s -- Copyright %s Nexteer',NxtrConf,first)
      | else
      |     fprintf('%s -- %s%s- %s Nexteer',NxtrConf,char(169),first,last)
      | end
  Data Store Write : DataStoreWrite  DataStoreName=NtcQlfr1
  Data Store Write1 : DataStoreWrite  DataStoreName=NtcQlfrHwAgOverTrvl
  Data Store Write2 : DataStoreWrite  DataStoreName=NtcStInfoHwAgOverTrvl
  Data Store Write3 : DataStoreWrite  DataStoreName=NtcStsHwAgOverTrvl
  Data Type Conversion : DataTypeConversion  OutDataTypeStr=Enum: SigQlfr1
  Data Type Conversion1 : DataTypeConversion  OutDataTypeStr=uint8
  Ground : Ground
  ISO Fault Debounce Design : Stateflow chart  TreatAsAtomicUnit=on
      settings: AttributesFormatString=|
      | Simulation Purpose Only.
      | Do Not Code this block
      | Diagnostic Manager Owns this requirement
  Terminator : Terminator
  Terminator1 : Terminator
  wires:
  NtcNr/1 -> Terminator/1
  DebStep/1 -> ISO Fault Debounce Design/2(DebStep)
  ISO Fault Debounce Design/1(Qualifier) -> Data Type Conversion/1
  Ground/1 -> ISO Fault Debounce Design/3(SvcClr)
  Data Type Conversion/1 -> Data Store Write1/1, Data Store Write/1
  NtcSts/1 -> Data Store Write3/1, ISO Fault Debounce Design/1(NtcSts)
  NtcStInfo/1 -> Data Type Conversion1/1, Terminator1/1
  Data Type Conversion1/1 -> Data Store Write2/1

== system SF011A_EotLrng/EotLrng/EotLrngPer1/HwAgCwAndCcwMax/CopyRight2 ==

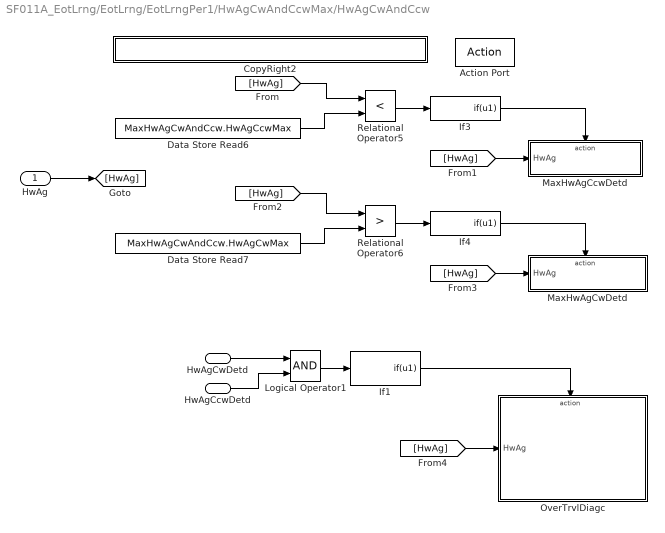
== system SF011A_EotLrng/EotLrng/EotLrngPer1/HwAgCwAndCcwMax/HwAgCwAndCcw ==
  HwAg : Inport  RequirementInfo={} %GIDa_c8cd5b7c_cbd1_476b_9743_899d5e4a1c86
  HwAgCwDetd : Inport  RequirementInfo={} %GIDa_8a24c917_6f4b_48d3_9c8e_402a340f61db  Port=2
  HwAgCcwDetd : Inport  RequirementInfo={} %GIDa_eafcbc20_c177_4872_bfb8_805f97224d01  Port=3
  Action Port : ActionPort  ActionType=then
  CopyRight2 : Subsystem  Description=|  mask(Copyright Information){none=on}
      | Copyright info block.                                               
      |                                                                     
      | Place copyright information at the top of every subsystem in design.
      mask prompts: none "No parameters"
      mask help: Place copyright information at the top of every subsystem in design.
      mask Display:
      | NxtrConf = 'Nexteer Confidential';
      | 
      | sys = bdroot; %handle for the current model ("system")
      | first = get_param(sys,'Created');
      | if(isempty(first))
      |     first = datestr(now,'yyyy');
      | else
      |     first = first(end-3:end);  %year is last four digits
      | end
      | 
      | last = get_param(sys,'LastModifiedDate');
      | if isempty(last)
      |     last = datestr(now,'yyyy');
      | else
      |     last = last(end-3:end);
      | end
      | 
      | if strcmp(first,last)
      |     fprintf('%s -- Copyright %s Nexteer',NxtrConf,first)
      | else
      |     fprintf('%s -- %s%s- %s Nexteer',NxtrConf,char(169),first,last)
      | end
  Data Store Read6 : DataStoreRead  RequirementInfo="{'linktype_rmi_doors' '0000ba59 (/E-STEER Core/SubSystem Specifications/Application Functions/SF011A Learned EOT Limits)' '#SF011A_156' 'true' 'REQ:  SF011A_156' '' } %GIDa_0cec739f_cedf_428b_b281_0fa530cc66c6"  DataStoreName=MaxHwAgCwAndCcw  DataStoreElements=MaxHwAgCwAndCcw.HwAgCcwMax
  Data Store Read7 : DataStoreRead  RequirementInfo="{'linktype_rmi_doors' '0000ba59 (/E-STEER Core/SubSystem Specifications/Application Functions/SF011A Learned EOT Limits)' '#SF011A_158' 'true' 'REQ:  SF011A_158' '' } %GIDa_2d25d9b4_6a5c_44c8_8b82_47be1f429b79"  DataStoreName=MaxHwAgCwAndCcw  DataStoreElements=MaxHwAgCwAndCcw.HwAgCwMax
  If1 : If  RequirementInfo="{'linktype_rmi_doors' '0000ba59 (/E-STEER Core/SubSystem Specifications/Application Functions/SF011A Learned EOT Limits)' '#SF011A_158' 'true' 'REQ:  SF011A_158' '' } %GIDa_892097bd_8db7_4641_aaa9_b8e55d260768"  IfExpression=u1  ShowElse=off
  If3 : If  RequirementInfo="{'linktype_rmi_doors' '0000ba59 (/E-STEER Core/SubSystem Specifications/Application Functions/SF011A Learned EOT Limits)' '#SF011A_156' 'true' 'REQ:  SF011A_156' '' } %GIDa_eff773a0_f378_4630_bbc3_9a1261b2e33a"  IfExpression=u1  ShowElse=off
  If4 : If  RequirementInfo="{'linktype_rmi_doors' '0000ba59 (/E-STEER Core/SubSystem Specifications/Application Functions/SF011A Learned EOT Limits)' '#SF011A_158' 'true' 'REQ:  SF011A_158' '' } %GIDa_ab57054b_8368_40b9_bbf8_6f3fe86d162f"  IfExpression=u1  ShowElse=off
  Logical Operator1 : Logic  RequirementInfo="{'linktype_rmi_doors' '0000ba59 (/E-STEER Core/SubSystem Specifications/Application Functions/SF011A Learned EOT Limits)' '#SF011A_158' 'true' 'REQ:  SF011A_158' '' } %GIDa_cc00eff5_b6b5_4e76_a489_f1d96f9e3e48"  AllPortsSameDT=off  OutDataTypeStr=boolean
  MaxHwAgCcwDetd : Subsystem  RequirementInfo="{'linktype_rmi_doors' '0000ba59 (/E-STEER Core/SubSystem Specifications/Application Functions/SF011A Learned EOT Limits)' '#SF011A_156' 'true' 'REQ:  SF011A_156' '' } %GIDa_435b5b2a_7f7d_4d0f_97d4_66841f6dd5f7"  TreatAsAtomicUnit=on
  MaxHwAgCwDetd : Subsystem  RequirementInfo="{'linktype_rmi_doors' '0000ba59 (/E-STEER Core/SubSystem Specifications/Application Functions/SF011A Learned EOT Limits)' '#SF011A_158' 'true' 'REQ:  SF011A_158' '' } %GIDa_3ea874a8_970d_45df_a46e_39c4dfcad9b4"  TreatAsAtomicUnit=on
  OverTrvlDiagc : Subsystem  TreatAsAtomicUnit=on
  Relational Operator5 : RelationalOperator  RequirementInfo="{'linktype_rmi_doors' '0000ba59 (/E-STEER Core/SubSystem Specifications/Application Functions/SF011A Learned EOT Limits)' '#SF011A_156' 'true' 'REQ:  SF011A_156' '' } %GIDa_df35c0dd_2824_4eec_a7e5_98745fcefb4a"  Operator=<  OutDataTypeStr=boolean
  Relational Operator6 : RelationalOperator  RequirementInfo="{'linktype_rmi_doors' '0000ba59 (/E-STEER Core/SubSystem Specifications/Application Functions/SF011A Learned EOT Limits)' '#SF011A_158' 'true' 'REQ:  SF011A_158' '' } %GIDa_33cc2a3b_d22f_4f0a_9175_c3826fdde7a9"  Operator=>  OutDataTypeStr=boolean
  wires:
  If3/1 -> MaxHwAgCcwDetd/Action
  Data Store Read6/1 -> Relational Operator5/2
  [HwAg] -> Relational Operator5/1
  [HwAg] -> MaxHwAgCcwDetd/1(HwAg)
  Relational Operator6/1 -> If4/1
  If4/1 -> MaxHwAgCwDetd/Action
  Relational Operator5/1 -> If3/1
  [HwAg] -> MaxHwAgCwDetd/1(HwAg)
  Data Store Read7/1 -> Relational Operator6/2
  [HwAg] -> Relational Operator6/1
  HwAg/1 -> [HwAg]
  HwAgCwDetd/1 -> Logical Operator1/1
  HwAgCcwDetd/1 -> Logical Operator1/2
  Logical Operator1/1 -> If1/1
  If1/1 -> OverTrvlDiagc/Action
  [HwAg] -> OverTrvlDiagc/1(HwAg)

== system SF011A_EotLrng/EotLrng/EotLrngPer1/SRLEna/ChkEotSigForNtc ==
  note: If ( Sig 0 and Sig 1 Available )
      | {
      | 	Perform correlation and In range check;
      | }
      | else
      | {
      | 	Set "Signal Available Fault" NTC;
      | }
  HwAgEotSig0Avl : Inport
  HwAgEotSig1Avl : Inport  Port=2
  HwAgEotSig0Cw : Inport  Port=3
  HwAgEotSig0Ccw : Inport  Port=4
  HwAgEotSig1Cw : Inport  Port=5
  HwAgEotSig1Ccw : Inport  Port=6
  Action Port : ActionPort  ActionType=then
  Constant1 : Constant  RequirementInfo={} %GIDa_52cae52c_bcf8_43ff_871f_ac660804e465  Value=DEBSTEP_CNT_U16
  Constant2 : Constant  RequirementInfo={} %GIDa_c4694c81_9589_4cb9_b92e_257094770507  Value=SIGAVLFLT_CNT_U08
  Constant3 : Constant  RequirementInfo={} %GIDa_79071866_041b_43ed_bc15_81fe8cf5f41c  Value=RackEotStorgFlt
  CopyRight2 : Subsystem  Description=|  mask(Copyright Information){none=on}
      | Copyright info block.                                               
      |                                                                     
      | Place copyright information at the top of every subsystem in design.
      mask prompts: none "No parameters"
      mask help: Place copyright information at the top of every subsystem in design.
      mask Display:
      | NxtrConf = 'Nexteer Confidential';
      | 
      | sys = bdroot; %handle for the current model ("system")
      | first = get_param(sys,'Created');
      | if(isempty(first))
      |     first = datestr(now,'yyyy');
      | else
      |     first = first(end-3:end);  %year is last four digits
      | end
      | 
      | last = get_param(sys,'LastModifiedDate');
      | if isempty(last)
      |     last = datestr(now,'yyyy');
      | else
      |     last = last(end-3:end);
      | end
      | 
      | if strcmp(first,last)
      |     fprintf('%s -- Copyright %s Nexteer',NxtrConf,first)
      | else
      |     fprintf('%s -- %s%s- %s Nexteer',NxtrConf,char(169),first,last)
      | end
  Enumerated Constant1 : simulink/Sources/Enumerated Constant  RequirementInfo={} %GIDa_bb824623_ecdf_44a1_8f01_2b74fcddf238  OutDataTypeStr=Enum: NtcSts1  Value=NtcSts1.NTCSTS_PREFAILD  SampleTime=inf
  EotSigAvl : Subsystem  TreatAsAtomicUnit=on
  If : If  RequirementInfo="{'linktype_rmi_doors' '0000ba59 (/E-STEER Core/SubSystem Specifications/Application Functions/SF011A Learned EOT Limits)' '#SF011A_145' 'true' 'REQ:  SF011A_145' '' } %GIDa_e06e6a97_1771_49b3_81a3_60749bee50ef"  NumInputs=2  IfExpression=u1 & u2
  SetSigAvlFltNtc : Subsystem  RequirementInfo="{'linktype_rmi_doors' '0000ba59 (/E-STEER Core/SubSystem Specifications/Application Functions/SF011A Learned EOT Limits)' '#SF011A_168' 'true' 'REQ:  SF011A_168' '' } %GIDa_4b3c4fca_6063_4e68_ad93_8d2689e87eff"  mask(SetNTC){}
      mask help: SetNTC library block
  wires:
  HwAgEotSig1Avl/1 -> If/2
  HwAgEotSig0Avl/1 -> If/1
  If/1 -> EotSigAvl/Action
  HwAgEotSig0Cw/1 -> EotSigAvl/1(HwAgEotSig0Cw)
  HwAgEotSig0Ccw/1 -> EotSigAvl/2(HwAgEotSig0Ccw)
  HwAgEotSig1Cw/1 -> EotSigAvl/3(HwAgEotSig1Cw)
  HwAgEotSig1Ccw/1 -> EotSigAvl/4(HwAgEotSig1Ccw)
  If/2 -> SetSigAvlFltNtc/Action
  Constant2/1 -> SetSigAvlFltNtc/2(NtcStInfo)
  Constant3/1 -> SetSigAvlFltNtc/1(NtcNr)
  Enumerated Constant1/1 -> SetSigAvlFltNtc/3(NtcSts)
  Constant1/1 -> SetSigAvlFltNtc/4(DebStep)

== system SF011A_EotLrng/EotLrng/EotLrngPer1/SRLEna/CopyRight2 ==

== system SF011A_EotLrng/EotLrng/EotLrngPer1/SRLEna/GetNtcQlfrSts ==
  NtcNr : Inport
  CopyRight2 : Subsystem  Description=|  mask(Copyright Information){none=on}
      | Copyright info block.                                               
      |                                                                     
      | Place copyright information at the top of every subsystem in design.
      mask prompts: none "No parameters"
      mask help: Place copyright information at the top of every subsystem in design.
      mask Display:
      | NxtrConf = 'Nexteer Confidential';
      | 
      | sys = bdroot; %handle for the current model ("system")
      | first = get_param(sys,'Created');
      | if(isempty(first))
      |     first = datestr(now,'yyyy');
      | else
      |     first = first(end-3:end);  %year is last four digits
      | end
      | 
      | last = get_param(sys,'LastModifiedDate');
      | if isempty(last)
      |     last = datestr(now,'yyyy');
      | else
      |     last = last(end-3:end);
      | end
      | 
      | if strcmp(first,last)
      |     fprintf('%s -- Copyright %s Nexteer',NxtrConf,first)
      | else
      |     fprintf('%s -- %s%s- %s Nexteer',NxtrConf,char(169),first,last)
      | end
  Data Store Read : DataStoreRead  DataStoreName=NtcQlfr
  Terminator : Terminator
  NtcQlfr : Outport
  wires:
  NtcNr/1 -> Terminator/1
  Data Store Read/1 -> NtcQlfr/1
